simulink model "RotorVirtualPlantModel_OpenLoop"  (R2022a)
settings: Solver=VariableStepAuto  StartTime=0.0  StopTime=10.0  RelTol=1e-3
values from neighbouring files (symbols this model uses):
  b = 0    [RotorSpeedControl.m]
  J_rotor = J_rodc+J_motor    (= 2.327e-05)    [RotorSpeedControl.m]
  K_m = 2.40E-2    (= 0.024)    [RotorSpeedControl.m]
  L = 0.23e-3    (= 0.00023)    [RotorSpeedControl.m]
  R = 3.85    [RotorSpeedControl.m]
  V_s = 12    [RotorSpeedControl.m]
settings Model: Creator=TC Tsao  LastModifiedBy=TC Tsao
settings SolverCC: AlgebraicLoopSolver=TrustRegion
settings DebuggingCC: UnconnectedInputMsg=warning  UnconnectedOutputMsg=warning  UnconnectedLineMsg=warning  SFMachineParentedDataDiag=warning
settings RTWCC: DLArmComputeVersion=19.05

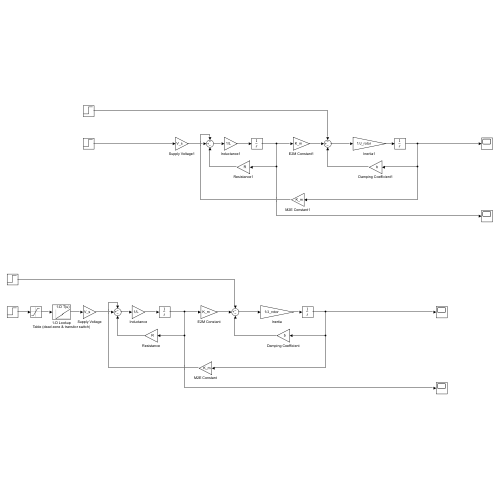
[thumbnail: Simulink's stored preview of the top-level diagram]
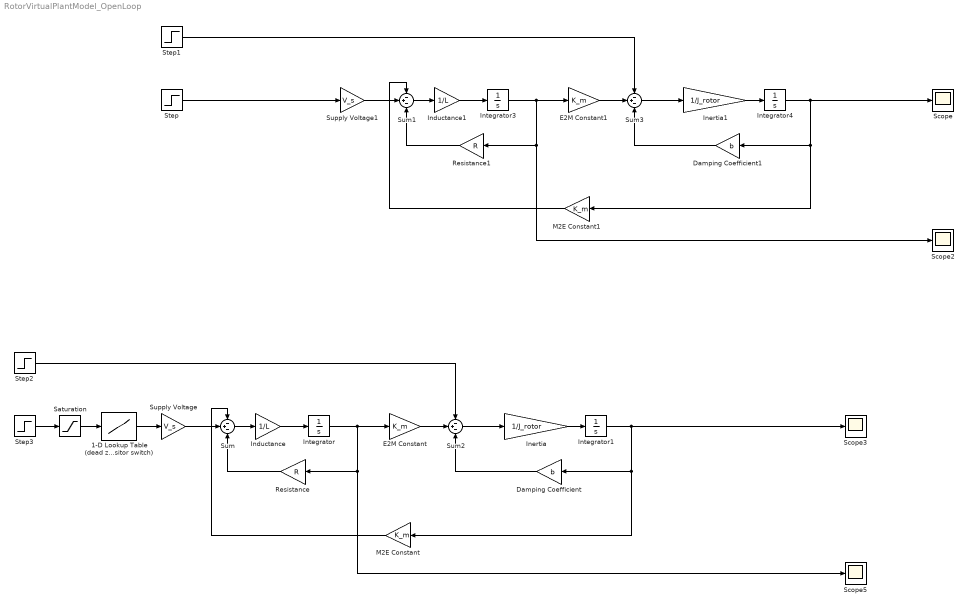
== system RotorVirtualPlantModel_OpenLoop ==
  1-D Lookup Table (dead zone & transitor switch) : Lookup_n-D  NumberOfTableDimensions=1  BreakpointsForDimension1=[-1,-0.96,-0.1,-0.06,-0.04,0,0.04,0.06,0.1,0.96,1]  Table=[-10.8,-10.8,-2,-1,-0,0,0,1,2,10.8,10.8]/V_s  InternalRulePriority=Speed  RndMeth=Simplest
  Damping Coefficient : Gain  Gain=b
  Damping Coefficient1 : Gain  Gain=b
  E2M Constant : Gain  Gain=K_m
  E2M Constant1 : Gain  Gain=K_m
  Inductance : Gain  Gain=1/L
  Inductance1 : Gain  Gain=1/L
  Inertia : Gain  Gain=1/J_rotor
  Inertia1 : Gain  Gain=1/J_rotor
  Integrator{,1,3..4} (4 alike) : Integrator
  M2E Constant : Gain  Gain=K_m
  M2E Constant1 : Gain  Gain=K_m
  Resistance : Gain  Gain=R
  Resistance1 : Gain  Gain=R
  Saturation : Saturate  UpperLimit=1  LowerLimit=-1
  Scope{,2..3,5} (4 alike) : Scope
  Step : Step  Time=0  SampleTime=0
  Step1 : Step  SampleTime=0
  Step2 : Step  SampleTime=0
  Step3 : Step  Time=0  SampleTime=0
  Sum{,1..3} (4 alike) : Sum  Inputs=-+-
  Supply Voltage : Gain  Gain=V_s
  Supply Voltage1 : Gain  Gain=V_s
  wires:
  Supply Voltage/1 -> Sum/2
  Sum2/1 -> Inertia/1
  Inertia/1 -> Integrator1/1
  Sum/1 -> Inductance/1
  Sum1/1 -> Inductance1/1
  M2E Constant1/1 -> Sum1/1
  Inductance1/1 -> Integrator3/1
  Integrator4/1 -> Scope/1, M2E Constant1/1, Damping Coefficient1/1
  Resistance/1 -> Sum/3
  Step2/1 -> Sum2/1
  Resistance1/1 -> Sum1/3
  E2M Constant1/1 -> Sum3/2
  Integrator/1 -> E2M Constant/1, Scope5/1, Resistance/1
  Saturation/1 -> 1-D Lookup Table (dead zone & transitor switch)/1
  M2E Constant/1 -> Sum/1
  Supply Voltage1/1 -> Sum1/2
  Damping Coefficient/1 -> Sum2/3
  Sum3/1 -> Inertia1/1
  Inertia1/1 -> Integrator4/1
  Integrator3/1 -> E2M Constant1/1, Scope2/1, Resistance1/1
  Inductance/1 -> Integrator/1
  Damping Coefficient1/1 -> Sum3/3
  Step1/1 -> Sum3/1
  1-D Lookup Table (dead zone & transitor switch)/1 -> Supply Voltage/1
  Integrator1/1 -> Scope3/1, M2E Constant/1, Damping Coefficient/1
  E2M Constant/1 -> Sum2/2
  Step/1 -> Supply Voltage1/1
  Step3/1 -> Saturation/1
